simulink library "BBCI_lib"  (Simulink 7.5)
settings: Solver=ode45  StartTime=0.0  StopTime=10.0  RelTol=1e-3
values from neighbouring files (symbols this model uses):
  pBBCI_kPa_AmbPSubVal_C = Simulink.Parameter    [BBCI_par.m]
  pBBCI_kPa_VacPres_CUR = Simulink.Parameter    [BBCI_par.m]
  pBBCI_mV_VacPresRaw_TAB = Simulink.Parameter    [BBCI_par.m]
libraries: BaseOperationLib_Browser x1, simulink x1
settings Model: Creator=wuaibin  LastModifiedBy=wuaibin

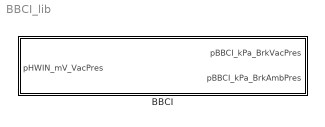
== system BBCI_lib ==
  BBCI : Subsystem  TreatAsAtomicUnit=on

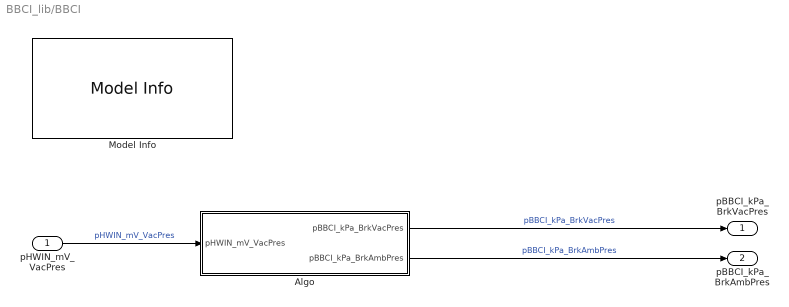
== system BBCI_lib/BBCI ==
  pHWIN_mV_VacPres : Inport  OutDataType=fixdt(1, 16)  OutScaling=2^0
  Algo : Subsystem
  Model Info : simulink/Model-Wide Utilities/Model Info  SystemSampleTime=-1  InitialBlockCM=None  BlockCM=None  Frame=on  DisplayStringWithTags=Model Info\nCreated: %<Created>\nCreator: wuaibin  HorizontalTextAlignment=Center  LeftAlignmentValue=0.5  SourceBlockDiagram=HQEV_HCU  TagMaxNumber=20
  pBBCI_kPa_BrkVacPres : Outport  OutDataType=fixdt(1, 16)  OutScaling=2^0
  pBBCI_kPa_BrkAmbPres : Outport  Port=2  OutDataType=fixdt(1, 16)  OutScaling=2^0
  wires:
  Algo/2(pBBCI_kPa_BrkAmbPres) -> pBBCI_kPa_BrkAmbPres/1  "pBBCI_kPa_BrkAmbPres"
  Algo/1(pBBCI_kPa_BrkVacPres) -> pBBCI_kPa_BrkVacPres/1  "pBBCI_kPa_BrkVacPres"
  pHWIN_mV_VacPres/1 -> Algo/1(pHWIN_mV_VacPres)  "pHWIN_mV_VacPres"

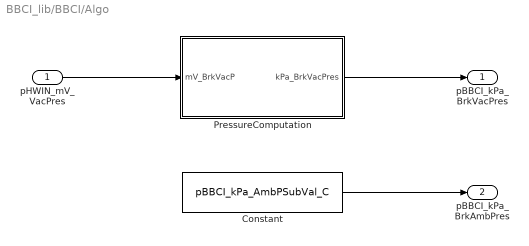
== system BBCI_lib/BBCI/Algo ==
  pHWIN_mV_VacPres : Inport  OutDataType=fixdt(1, 16)  OutScaling=2^0
  Constant : Constant  Value=pBBCI_kPa_AmbPSubVal_C  OutDataType=fixdt(1, 16)  OutScaling=2^0  OutDataTypeStr=Inherit: Inherit via back propagation
      mask Display: patch([0 1 1 1 .75], [1 1 0 .75 1], [0 1 0]);
  PressureComputation : Subsystem
  pBBCI_kPa_BrkVacPres : Outport  OutDataType=fixdt(1, 16)  OutScaling=2^0
  pBBCI_kPa_BrkAmbPres : Outport  Port=2  OutDataType=fixdt(1, 16)  OutScaling=2^0
  wires:
  Constant/1 -> pBBCI_kPa_BrkAmbPres/1
  PressureComputation/1(kPa_BrkVacPres) -> pBBCI_kPa_BrkVacPres/1
  pHWIN_mV_VacPres/1 -> PressureComputation/1(mV_BrkVacP)

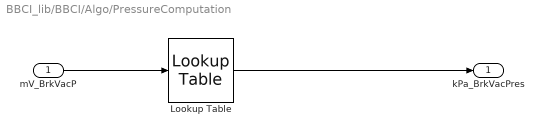
== system BBCI_lib/BBCI/Algo/PressureComputation ==
  mV_BrkVacP : Inport
  Lookup Table : BaseOperationLib_Browser/Lookup Tables Changed/Lookup Table  InputValues=pBBCI_mV_VacPresRaw_TAB  Table=pBBCI_kPa_VacPres_CUR  LookUpMeth=Interpolation-Use End Values  OutMin=[]  OutMax=[]  OutDataType=fixdt(1, 16)  OutScaling=2^0  OutDataTypeStr=Inherit: Inherit via back propagation  SaturateOnIntegerOverflow=on
      settings: AttributesFormatString=X:%<InputValues>\nTAB:%<Table>
  kPa_BrkVacPres : Outport
  wires:
  Lookup Table/1 -> kPa_BrkVacPres/1
  mV_BrkVacP/1 -> Lookup Table/1
